simulink model "Road monito-2024r"  (R2021a)
settings: Solver=FixedStepDiscrete  StartTime=0.0  StopTime=inf  FixedStep=0.1  RelTol=1e-3
libraries: simulink x29
(part 2 of 2)

== system Road monito-2024r/rule81_2 ==
  light : Inport
  Enable : EnablePort  StatesWhenEnabling=reset
  light usage : MATLAB Function  TreatAsAtomicUnit=on
  y : Outport  OutputWhenDisabled=reset  InitialOutput=0
  wires:
  light usage/1(y) -> y/1
  light/1 -> light usage/1(light)

== system Road monito-2024r/rule81_3 ==
  Ego : Inport
  Enable : EnablePort  StatesWhenEnabling=reset
  Speedmonitor : MATLAB Function  TreatAsAtomicUnit=on
  y1 : Outport  OutputWhenDisabled=reset  InitialOutput=0
  cs : Outport  Port=2  OutputWhenDisabled=reset  InitialOutput=[0 120]
  wires:
  Speedmonitor/2(cs) -> cs/1
  Ego/1 -> Speedmonitor/1(Ego)
  Speedmonitor/1(y) -> y1/1

== system Road monito-2024r/rule81_4 ==
  Ego : Inport
  Enable : EnablePort  StatesWhenEnabling=reset
  Speedmonitor : MATLAB Function  TreatAsAtomicUnit=on
  y1 : Outport  OutputWhenDisabled=reset  InitialOutput=0
  cs : Outport  Port=2  OutputWhenDisabled=reset  InitialOutput=[0 120]
  wires:
  Speedmonitor/2(cs) -> cs/1
  Ego/1 -> Speedmonitor/1(Ego)
  Speedmonitor/1(y) -> y1/1

== system Road monito-2024r/rule81_5 ==
  Ego : Inport
  Enable : EnablePort  StatesWhenEnabling=reset
  Speedmonitor : MATLAB Function  TreatAsAtomicUnit=on
  y1 : Outport  OutputWhenDisabled=reset  InitialOutput=0
  cs : Outport  Port=2  OutputWhenDisabled=reset  InitialOutput=[0 120]
  wires:
  Speedmonitor/2(cs) -> cs/1
  Ego/1 -> Speedmonitor/1(Ego)
  Speedmonitor/1(y) -> y1/1

== system Road monito-2024r/rule81_6 ==
  Enable : EnablePort  StatesWhenEnabling=reset
  Constant : Constant  Value=100
  CD : Outport  OutputWhenDisabled=reset  InitialOutput=-1
  wires:
  Constant/1 -> CD/1

== system Road monito-2024r/rule81_7 ==
  Enable : EnablePort  StatesWhenEnabling=reset
  Constant : Constant  Value=50
  CD : Outport  OutputWhenDisabled=reset  InitialOutput=-1
  wires:
  Constant/1 -> CD/1

== system Road monito-2024r/rule82_1 ==
  Ego : Inport
  Enable : EnablePort  StatesWhenEnabling=reset
  Speedmonitor : MATLAB Function  TreatAsAtomicUnit=on
  y1 : Outport  OutputWhenDisabled=reset  InitialOutput=0
  wires:
  Ego/1 -> Speedmonitor/1(Ego)
  Speedmonitor/1(y) -> y1/1

== system Road monito-2024r/rule82_2 ==
  decision : Inport
  left1 : Inport  Port=2
  Enable : EnablePort  StatesWhenEnabling=reset
  Compare To Constant : simulink/Logic and Bit Operations/Compare To Constant  relop===  const=6  OutDataTypeStr=boolean
  Logical Operator : Logic  AllPortsSameDT=off  OutDataTypeStr=boolean
  y1 : Outport  OutputWhenDisabled=reset  InitialOutput=0
  wires:
  decision/1 -> Compare To Constant/1
  Compare To Constant/1 -> Logical Operator/1
  left1/1 -> Logical Operator/2
  Logical Operator/1 -> y1/1

== system Road monito-2024r/rule82_3 ==
  note: 待开发
  Enable : EnablePort  StatesWhenEnabling=reset
  Constant : Constant  Value=0
  y1 : Outport  OutputWhenDisabled=reset  InitialOutput=0
  wires:
  Constant/1 -> y1/1

== system Road monito-2024r/rule82_4 ==
  Ego : Inport
  Enable : EnablePort  StatesWhenEnabling=reset
  Speedmonitor : MATLAB Function  TreatAsAtomicUnit=on
  y1 : Outport  OutputWhenDisabled=reset  InitialOutput=0
  wires:
  Ego/1 -> Speedmonitor/1(Ego)
  Speedmonitor/1(y) -> y1/1

== system Road monito-2024r/rule82_5 ==
  overlap : Inport
  Enable : EnablePort  StatesWhenEnabling=reset
  Constant : Constant
  Constant1 : Constant  Value=0
  Switch : Switch  Criteria=u2 > Threshold
  y1 : Outport  OutputWhenDisabled=reset  InitialOutput=0
  wires:
  overlap/1 -> Switch/2
  Constant/1 -> Switch/1
  Constant1/1 -> Switch/3
  Switch/1 -> y1/1

== system Road monito-2024r/rule_47_2_2 ==
  T1_2_2 : Inport
  t1_2_4 : Inport  Port=2
  Ego : Inport  Port=3
  Tgtrf : Inport  Port=4
  Tgtrr : Inport  Port=5
  Enable : EnablePort  StatesWhenEnabling=reset
  Logical Operator : Logic  Operator=OR  AllPortsSameDT=off  OutDataTypeStr=boolean
  MATLAB Function : MATLAB Function  TreatAsAtomicUnit=on
  MATLAB Function1 : MATLAB Function  TreatAsAtomicUnit=on
  Out1 : Outport  OutputWhenDisabled=reset  InitialOutput=0
  wires:
  T1_2_2/1 -> MATLAB Function/1(t122)
  Ego/1 -> MATLAB Function1/2(Ego), MATLAB Function/2(Ego)
  Tgtrf/1 -> MATLAB Function/3(Tgtrf)
  t1_2_4/1 -> MATLAB Function1/1(t124)
  Tgtrr/1 -> MATLAB Function1/3(Tgtrr)
  MATLAB Function/1(y) -> Logical Operator/1
  MATLAB Function1/1(y) -> Logical Operator/2
  Logical Operator/1 -> Out1/1

== system Road monito-2024r/rule_dis ==
  Tgt_f : Inport
  Ego : Inport  Port=2
  Ego_fl : Inport  Port=3
  ycd : Inport  Port=4
  Enable : EnablePort  StatesWhenEnabling=reset
  FollowingDistance : MATLAB Function  TreatAsAtomicUnit=on
  y : Outport  OutputWhenDisabled=reset  InitialOutput=0
  wires:
  Tgt_f/1 -> FollowingDistance/2(Tgt_f)
  FollowingDistance/1(y) -> y/1
  Ego/1 -> FollowingDistance/1(Ego)
  Ego_fl/1 -> FollowingDistance/3(Ego_fl)
  ycd/1 -> FollowingDistance/4(ycd)

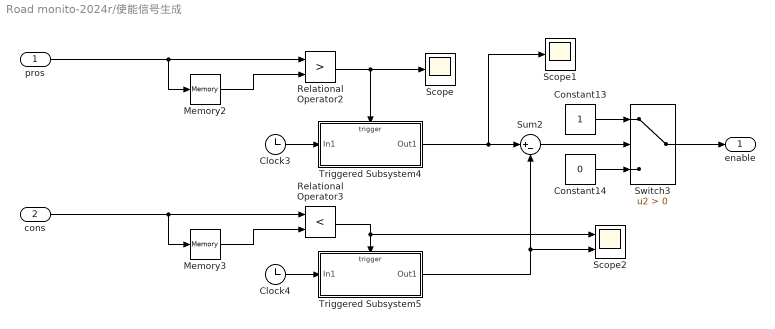
== system Road monito-2024r/使能信号生成 ==
  pros : Inport
  cons : Inport  Port=2
  Clock3 : Clock
  Clock4 : Clock
  Constant13 : Constant
  Constant14 : Constant  Value=0
  Memory2 : Memory
  Memory3 : Memory
  Relational Operator2 : RelationalOperator  Operator=>  OutDataTypeStr=boolean  RndMeth=Simplest
  Relational Operator3 : RelationalOperator  Operator=<  OutDataTypeStr=boolean  RndMeth=Simplest
  Scope : Scope
  Scope1 : Scope
  Scope2 : Scope  NumInputPorts=2
  Sum2 : Sum  Inputs=|+-
  Switch3 : Switch  Criteria=u2 > Threshold
  Triggered Subsystem4 : Subsystem  TreatAsAtomicUnit=on
  Triggered Subsystem5 : Subsystem  TreatAsAtomicUnit=on
  enable : Outport
  wires:
  Relational Operator3/1 -> Triggered Subsystem5/Trigger, Scope2/1
  Constant14/1 -> Switch3/3
  Triggered Subsystem4/1(Out1) -> Scope1/1, Sum2/1
  Sum2/1 -> Switch3/2
  pros/1 -> Memory2/1, Relational Operator2/1
  Clock4/1 -> Triggered Subsystem5/1(In1)
  Memory3/1 -> Relational Operator3/2
  Relational Operator2/1 -> Scope/1, Triggered Subsystem4/Trigger
  Memory2/1 -> Relational Operator2/2
  Clock3/1 -> Triggered Subsystem4/1(In1)
  Triggered Subsystem5/1(Out1) -> Scope2/2, Sum2/2
  Constant13/1 -> Switch3/1
  Switch3/1 -> enable/1
  cons/1 -> Memory3/1, Relational Operator3/1

== system Road monito-2024r/Enabled Subsystem/Triggered Subsystem2 ==
  In1 : Inport
  Trigger : TriggerPort  VariantControl=Variant
  Output : Outport  InitialOutput=0  VectorParamsAs1DForOutWhenUnconnected=off
  wires:
  In1/1 -> Output/1

== system Road monito-2024r/Enabled Subsystem1/Triggered Subsystem2 ==
  In1 : Inport
  Trigger : TriggerPort  VariantControl=Variant
  Output : Outport  InitialOutput=0  VectorParamsAs1DForOutWhenUnconnected=off
  wires:
  In1/1 -> Output/1

== system Road monito-2024r/Subsystem2/Enabled Subsystem1 ==
  t2_out : Inport
  roadinfo : Inport  Port=2
  Enable : EnablePort
  Selector1 : Selector  InputPortWidth=3  IndexOptions=Index vector (dialog)  Indices=[2]  OutputSizes=1
  t2 : Outport  InitialOutput=-10
  t2_laneid : Outport  Port=2  InitialOutput=0
  wires:
  t2_out/1 -> t2/1  "上一次下降沿时间"
  roadinfo/1 -> Selector1/1
  Selector1/1 -> t2_laneid/1  "上一次下降沿所在的车道"

== system Road monito-2024r/Subsystem2/Triggered Subsystem1 ==
  t1_out : Inport
  t_now : Inport  Port=2
  laneinfo : Inport  Port=3
  Trigger : TriggerPort  VariantControl=(inherit)
  t1 : Outport  InitialOutput=-20
  t3 : Outport  Port=2  InitialOutput=-10
  t1_lanid : Outport  Port=3  InitialOutput=0
  wires:
  t1_out/1 -> t1/1  "上一次上升沿时间"
  t_now/1 -> t3/1  "这一次上升沿时间"
  laneinfo/1 -> t1_lanid/1  "上一次上升沿时所在的车道"

== system Road monito-2024r/Timing module/Triggered Subsystem1 ==
  In1 : Inport
  In2 : Inport  Port=2
  Trigger : TriggerPort  TriggerType=falling  VariantControl=Variant
  Add : Sum  Inputs=-+
  Out1 : Outport  VectorParamsAs1DForOutWhenUnconnected=off
  wires:
  Add/1 -> Out1/1
  In2/1 -> Add/2
  In1/1 -> Add/1

== system Road monito-2024r/Timing module/Triggered Subsystem2 ==
  In1 : Inport
  Trigger : TriggerPort  VariantControl=Variant
  Out1 : Outport  InitialOutput=0  VectorParamsAs1DForOutWhenUnconnected=off
  wires:
  In1/1 -> Out1/1

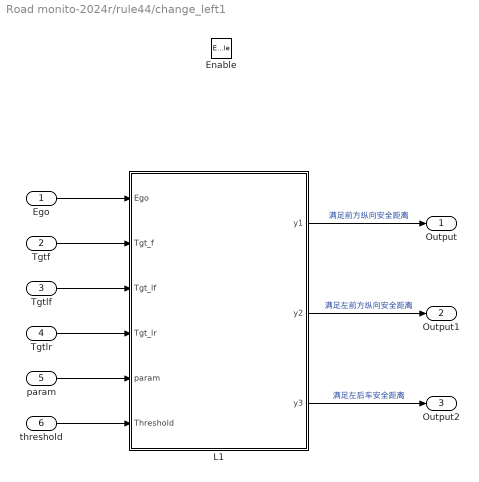
== system Road monito-2024r/rule44/change_left1 ==
  Ego : Inport
  Tgtf : Inport  Port=2
  Tgtlf : Inport  Port=3
  Tgtlr : Inport  Port=4
  param : Inport  Port=5
  threshold : Inport  Port=6
  Enable : EnablePort  StatesWhenEnabling=reset
  L1 : MATLAB Function  TreatAsAtomicUnit=on
  Output : Outport  OutputWhenDisabled=reset  InitialOutput=0
  Output1 : Outport  Port=2  OutputWhenDisabled=reset  InitialOutput=0
  Output2 : Outport  Port=3  OutputWhenDisabled=reset  InitialOutput=0
  wires:
  Ego/1 -> L1/1(Ego)
  Tgtf/1 -> L1/2(Tgt_f)
  Tgtlf/1 -> L1/3(Tgt_lf)
  Tgtlr/1 -> L1/4(Tgt_lr)
  param/1 -> L1/5(param)
  threshold/1 -> L1/6(Threshold)
  L1/1(y1) -> Output/1  "满足前方纵向安全距离"
  L1/2(y2) -> Output1/1  "满足左前方纵向安全距离"
  L1/3(y3) -> Output2/1  "满足左后车安全距离"

== system Road monito-2024r/rule44/change_left2 ==
  Ego : Inport
  Tgtf : Inport  Port=2
  Tgtr : Inport  Port=3
  param : Inport  Port=4
  threshold : Inport  Port=5
  Enable : EnablePort  StatesWhenEnabling=reset
  beforerchangelane : MATLAB Function  TreatAsAtomicUnit=on
  Output1 : Outport  OutputWhenDisabled=reset  InitialOutput=0
  Output2 : Outport  Port=2  OutputWhenDisabled=reset  InitialOutput=0
  wires:
  Ego/1 -> beforerchangelane/3(Ego)
  Tgtf/1 -> beforerchangelane/1(Tgt_f)
  Tgtr/1 -> beforerchangelane/2(Tgt_r)
  param/1 -> beforerchangelane/4(param)
  threshold/1 -> beforerchangelane/5(Threshold)
  beforerchangelane/1(y2) -> Output1/1  "满足前方纵向安全距离"
  beforerchangelane/2(y3) -> Output2/1  "满足后车安全距离"

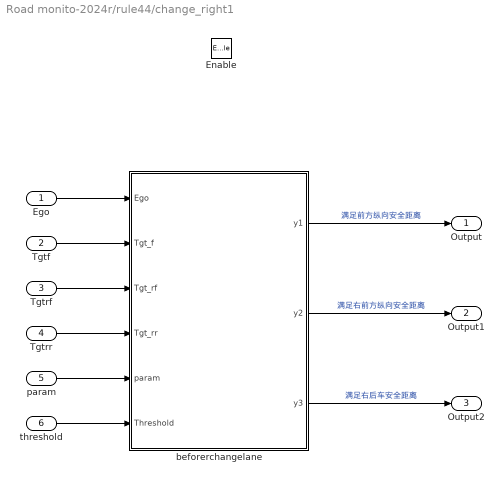
== system Road monito-2024r/rule44/change_right1 ==
  Ego : Inport
  Tgtf : Inport  Port=2
  Tgtrf : Inport  Port=3
  Tgtrr : Inport  Port=4
  param : Inport  Port=5
  threshold : Inport  Port=6
  Enable : EnablePort  StatesWhenEnabling=reset
  beforerchangelane : MATLAB Function  TreatAsAtomicUnit=on
  Output : Outport  OutputWhenDisabled=reset  InitialOutput=0
  Output1 : Outport  Port=2  OutputWhenDisabled=reset  InitialOutput=0
  Output2 : Outport  Port=3  OutputWhenDisabled=reset  InitialOutput=0
  wires:
  Ego/1 -> beforerchangelane/1(Ego)
  Tgtf/1 -> beforerchangelane/2(Tgt_f)
  Tgtrf/1 -> beforerchangelane/3(Tgt_rf)
  Tgtrr/1 -> beforerchangelane/4(Tgt_rr)
  param/1 -> beforerchangelane/5(param)
  threshold/1 -> beforerchangelane/6(Threshold)
  beforerchangelane/1(y1) -> Output/1  "满足前方纵向安全距离"
  beforerchangelane/2(y2) -> Output1/1  "满足右前方纵向安全距离"
  beforerchangelane/3(y3) -> Output2/1  "满足右后车安全距离"

== system Road monito-2024r/rule44/change_right2 ==
  Ego : Inport
  Tgtf : Inport  Port=2
  Tgtr : Inport  Port=3
  param : Inport  Port=4
  threshold : Inport  Port=5
  Enable : EnablePort  StatesWhenEnabling=reset
  beforerchangelane : MATLAB Function  TreatAsAtomicUnit=on
  Output1 : Outport  OutputWhenDisabled=reset  InitialOutput=0
  Output2 : Outport  Port=2  OutputWhenDisabled=reset  InitialOutput=0
  wires:
  Ego/1 -> beforerchangelane/3(Ego)
  Tgtf/1 -> beforerchangelane/1(Tgt_f)
  Tgtr/1 -> beforerchangelane/2(Tgt_r)
  param/1 -> beforerchangelane/4(param)
  threshold/1 -> beforerchangelane/5(Threshold)
  beforerchangelane/1(y2) -> Output1/1  "满足前方纵向安全距离"
  beforerchangelane/2(y3) -> Output2/1  "满足后车安全距离"

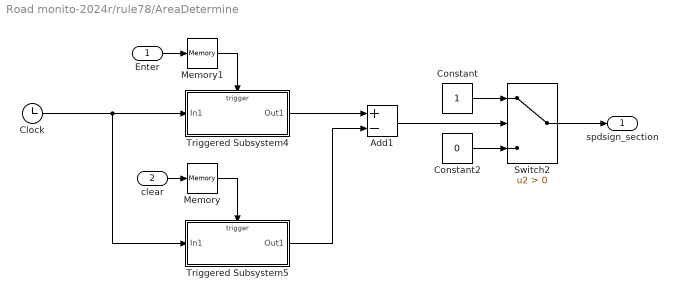
== system Road monito-2024r/rule78/AreaDetermine ==
  Enter : Inport
  clear : Inport  Port=2
  Add1 : Sum  Inputs=+-
  Clock : Clock
  Constant : Constant
  Constant2 : Constant  Value=0
  Memory : Memory
  Memory1 : Memory
  Switch2 : Switch  Criteria=u2 > Threshold
  Triggered Subsystem4 : Subsystem  TreatAsAtomicUnit=on
  Triggered Subsystem5 : Subsystem  TreatAsAtomicUnit=on
  spdsign_section : Outport
  wires:
  Triggered Subsystem4/1(Out1) -> Add1/1
  Enter/1 -> Memory1/1
  Switch2/1 -> spdsign_section/1
  clear/1 -> Memory/1
  Triggered Subsystem5/1(Out1) -> Add1/2
  Add1/1 -> Switch2/2
  Constant2/1 -> Switch2/3
  Memory/1 -> Triggered Subsystem5/Trigger
  Clock/1 -> Triggered Subsystem4/1(In1), Triggered Subsystem5/1(In1)
  Constant/1 -> Switch2/1
  Memory1/1 -> Triggered Subsystem4/Trigger

== system Road monito-2024r/使能信号生成/Triggered Subsystem4 ==
  In1 : Inport
  Trigger : TriggerPort  TriggerType=either  VariantControl=(inherit)
  Out1 : Outport
  wires:
  In1/1 -> Out1/1

== system Road monito-2024r/使能信号生成/Triggered Subsystem5 ==
  In1 : Inport
  Trigger : TriggerPort  VariantControl=(inherit)
  Out1 : Outport
  wires:
  In1/1 -> Out1/1

== system Road monito-2024r/rule78/AreaDetermine/Triggered Subsystem4 ==
  In1 : Inport
  Trigger : TriggerPort  VariantControl=(inherit)
  Out1 : Outport
  wires:
  In1/1 -> Out1/1

== system Road monito-2024r/rule78/AreaDetermine/Triggered Subsystem5 ==
  In1 : Inport
  Trigger : TriggerPort  VariantControl=(inherit)
  Out1 : Outport
  wires:
  In1/1 -> Out1/1

== matlab function Road monito-2024r/rule80/FollowingDistance ==
  data: Ego input; CD output
function CD = fcn(Ego)
%参数需求
Egovx = Ego(4);                   %自车纵向速度(m/s)

if Egovx >= 100/3.6
    CD = 100;
else
    CD = 50;
end

== matlab function Road monito-2024r/rule44/MATLAB Function ==
  data: u input; y output
function y = fcn(u)

if u == 0
    y = 0;
elseif u == 1
    y = 44.22;
elseif u == 2
    y = 44.23;
elseif u == 3
    y = 44.24;
else
    y = 0;
end

== matlab function Road monito-2024r/rule44/MATLAB Function1 ==
  data: u input; y output
function y = fcn(u)

if u == 0
    y = 0;
elseif u == 1
    y = 44.25;
elseif u == 2
    y = 44.26;
elseif u == 3
    y = 44.27;
else
    y = 0;
end

== matlab function Road monito-2024r/rule44/MATLAB Function2 ==
  data: u input; y output
function y = fcn(u)

if u == 0
    y = 0;
elseif u == 1
    y = 44.12;
elseif u == 2
    y = 44.13;
elseif u == 3
    y = 44.14;
else
    y = 0;
end

== matlab function Road monito-2024r/T_rule78 ==
  data: roadinfo input; y output
function y = fcn(roadinfo)
if roadinfo(1)==1
    y = 1;
else
    y = 0;
end

== matlab function Road monito-2024r/rule78/Speedsigncalculate ==
  data: Enter_spdlimit_section output; Ego input; speedsign input
function Enter_spdlimit_section = fcn(Ego,speedsign)
%%

%参数需求
s_speedsign = speedsign(1);         %限速标志位置(m)(感知范围内无标志则输入为2000）
Egox = Ego(1);
%高速主路限速条件判断
if s_speedsign < Egox       %限速标志检测，只用于判断是否进入限速标志管理区域
    Enter_spdlimit_section = 1;
else
    Enter_spdlimit_section = 0;
end

== matlab function Road monito-2024r/rule78/Speedmonitor ==
  data: Ego input; speedsign input; respeedsign input; spdsign_section input; y output; cs output; clear output; roadinfo input
function [y,cs,clear] = fcn(Ego,speedsign,respeedsign,spdsign_section,roadinfo)
%%

%参数需求
Ego_x = Ego(1);
Ego_vx = Ego(4);
vxmax_speedsign = speedsign(3);     %限速标志限制的速度上限(km/h)
vxmin_speedsign = speedsign(4);     %限速标志限制的速度下限(km/h)（无则输入为60）
s_releasespdsign = respeedsign(1);  %解除限速标志位置(m)(无则输入为0）
roadid = roadinfo(2);
roadnum = roadinfo(3);

%高速主路限速触发条件判断
if spdsign_section == 1       %自车处于限速标志管理路段
    if Ego_vx >= vxmin_speedsign/3.6 && Ego_vx <= vxmax_speedsign/3.6
        y = 0;
    else
        y = 1;
    end
    cs = [vxmin_speedsign vxmax_speedsign];
else                         %自车处于非限速标志管理路段
    if roadnum==2 && roadid==1
        if Ego_vx >= 100/3.6 && Ego_vx <= 120/3.6
            y = 0;
        else
            y = 1;
        end
        cs = [100 120];
    elseif roadnum>=3 && roadid==1
        if Ego_vx >= 110/3.6 && Ego_vx <= 120/3.6
            y = 0;
        else
            y = 1;
        end
        cs = [110 120];
    elseif roadnum>=3 && roadid>1 && roadid<roadnum
        if Ego_vx >= 90/3.6 && Ego_vx <= 120/3.6
            y = 0;
        else
            y = 1;
        end
        cs = [90 120];
    else
        y = 0;
        cs = [60 100];
    end
end
if s_releasespdsign < Ego_x           %解除限速标志位置，用于反馈确定自车所在区域
    clear = 1;
else
    clear = 0;
end

== matlab function Road monito-2024r/rule44/MATLAB Function3 ==
  data: u input; y output
function y = fcn(u)

if u == 0
    y = 0;
elseif u == 1
    y = 44.15;
elseif u == 2
    y = 44.16;
elseif u == 3
    y = 44.17;
else
    y = 0;
end

== matlab function Road monito-2024r/T_rule46_1 ==
  data: env input; y1 output; y2 output; y3 output
function [y1,y2,y3] = fcn(env)
if env(1)<50
    y1 = true;
    y2 = false;
    y3 = false;
elseif env(1)<100
    y1 = false;
    y2 = true;
    y3 = false;
elseif env(1)<200
    y1 = false;
    y2 = false;
    y3 = true;
else
    y1 = false;
    y2 = false;
    y3 = false;
end

== matlab function Road monito-2024r/rule46_1/Speedmonitor ==
  data: Ego input; y output; cs output
function [y,cs] = fcn(Ego)
%%

%参数需求
Ego_vx = Ego(4);


if Ego_vx <= 30/3.6
    y = 0;
else
    y = 1;
end
cs = [0 30];

== matlab function Road monito-2024r/T_rule46_2 ==
  data: env input; y output
function y = fcn(env)
if env(2)==1
    y = 1;
else
    y = 0;
end

== matlab function Road monito-2024r/rule46_2/Speedmonitor ==
  data: Ego input; y output; cs output
function [y,cs] = fcn(Ego)
%%

%参数需求
Ego_vx = Ego(4);


if Ego_vx <= 30/3.6
    y = 0;
else
    y = 1;
end
cs = [0 30];

== matlab function Road monito-2024r/rule44/change_right1/beforerchangelane ==
  data: Ego input; Tgt_f input; Tgt_rf input; Tgt_rr input; y1 output; y2 output; y3 output; param input; Threshold input
function [y1,y2,y3] = fcn(Ego,Tgt_f,Tgt_rf,Tgt_rr,param,Threshold)
%%

%参数需求

Tgtx_rr = Tgt_rr(1);             
Tgty_rr = Tgt_rr(2);              
Tgtvx_rr = Tgt_rr(3);
Tgtl_rr = Tgt_rr(5);
Egox = Ego(1);
Egovx = Ego(4);
Egol = param(1);
Ego_fl = param(3);
Tgtx_f = Tgt_f(1);              
Tgty_f = Tgt_f(2);
Tgtvx_f = Tgt_f(3);
Tgtl_f = Tgt_f(5);
Tgtx_rf = Tgt_rf(1);              
Tgty_rf = Tgt_rf(2);
Tgtvx_rf = Tgt_rf(3); 
Tgtl_rf = Tgt_rf(5);
dclmin = Threshold(9) * (Egovx - Tgtvx_rr) + Threshold(10);         %最小换道距离
if dclmin > 50
    dclmin = 50;
elseif dclmin < 0
    dclmin = 0;
else
    dclmin = dclmin;
end
TTCx = Threshold(3);           %安全碰撞时间

%与前车的安全距离判断
if Tgtx_f == 2000 && Tgty_f == 2000       %坐标为2000视为不存在前车
    y1 = 0;   
else
    if Tgtx_f-Egox-0.5*Tgtl_f-Ego_fl < (Egovx - Tgtvx_f) * TTCx 
        y1 = 1;
%     elseif Tgtx_f-Egox-0.5*Tgtl_f-Ego_fl < dclmin %前车暂不考虑车距
%         y1 = 2;
    else
        y1 = 0;
    end
end
%与右前车的安全距离判断
if Tgtx_rf == 2000 && Tgty_rf == 2000     %坐标为2000视为不存在右前车
    y2 = 0;
else
    if Tgtx_rf-Egox-0.5*Tgtl_rf-Ego_fl < (Egovx - Tgtvx_rf) * TTCx 
        y2 = 1;
    else
        y2 = 0;
    end
end
%与右后车的安全距离判断
if Tgtx_rr == 2000 && Tgty_rr == 2000   %坐标为2000视为不存在右后车
    y3 = 0;
else
    if Egox-Tgtx_rr-0.5*Tgtl_rr-(Egol-Ego_fl) < dclmin
        y3 = 3;
    else
        y3 = 0;
    end
end

== matlab function Road monito-2024r/rule47_1_l/Speedmonitor ==
  data: threshold input; light input; y output
function y = fcn(threshold,light)
%%
t_cl = threshold(4);

if light >= t_cl
    y = 0;
else
    y = 1;
end

== matlab function Road monito-2024r/rule47_1_r/Speedmonitor ==
  data: threshold input; light input; y output
function y = fcn(threshold,light)
%%
t_cl = threshold(4);

if light >= t_cl
    y = 0;
else
    y = 1;
end

== matlab function Road monito-2024r/rule1_43/MATLAB Function ==
  data: Tgtf input; y output; left input
function y = fcn(Tgtf,left)

Tgtfx = Tgtf(1);
Tgtfy = Tgtf(2);
Tgtfvy = Tgtf(4);
Tgtfw = Tgtf(6);

yTgt_l = Tgtfy + 0.5 * Tgtfw;
yTgt_r = Tgtfy - 0.5 * Tgtfw;

Y_leftline_Ego = polyval(left(2:end-1),Tgtfx);

if Y_leftline_Ego<yTgt_l && Y_leftline_Ego>yTgt_r
    y1 = 1;
else
    y1 = 0;
end

if Tgtfvy > 0.2
    y2 = 1;
else
    y2 = 0;
end

if y1==1 && y2 ==1
    y = 1;
else
    y = 0;
end

== matlab function Road monito-2024r/T_overlapline ==
  data: param input; left input; right input; y output
function y = fcn(param,left,right)

Ego_l = param(1);
Ego_w = param(2);
Ego_fl = param(3);

yEgo_lf = 0.5 * Ego_w;
yEgo_rf = -0.5 * Ego_w;
yEgo_lr = 0.5 * Ego_w;
yEgo_rr = -0.5 * Ego_w;

Y_leftline_Egof = polyval(left(2:end-1),Ego_fl);
Y_leftline_Egor = polyval(left(2:end-1),Ego_fl - Ego_l);
Y_rightline_Egof = polyval(right(2:end-1),Ego_fl);
Y_rightline_Egor = polyval(right(2:end-1),Ego_fl - Ego_l);

if Y_leftline_Egof<yEgo_lf && Y_leftline_Egof>yEgo_rf
    y = 1;
elseif Y_rightline_Egof<yEgo_lf && Y_rightline_Egof>yEgo_rf
    y = 2;
elseif Y_leftline_Egor<yEgo_lr && Y_leftline_Egor>yEgo_rr
    y = 1;
elseif Y_rightline_Egor<yEgo_lr && Y_rightline_Egor>yEgo_rr
    y = 2;
else
    y = 0;
end

== matlab function Road monito-2024r/rule1_43/MATLAB Function1 ==
  data: Tgtlf input; y output; left input
function y = fcn(Tgtlf,left)

Tgtlfx = Tgtlf(1);
Tgtlfy = Tgtlf(2);
Tgtlfvy = Tgtlf(4);
Tgtlfw = Tgtlf(6);

yTgt_l = Tgtlfy + 0.5 * Tgtlfw;
yTgt_r = Tgtlfy - 0.5 * Tgtlfw;

Y_leftline_Ego = polyval(left(2:end-1),Tgtlfx);

if Y_leftline_Ego<yTgt_l && Y_leftline_Ego>yTgt_r
    y1 = 1;
else
    y1 = 0;
end

if Tgtlfvy > 0.2
    y2 = 1;
else
    y2 = 0;
end

if y1==1 && y2 ==1
    y = 1;
else
    y = 0;
end

== matlab function Road monito-2024r/rule_47_2_2/MATLAB Function ==
  data: t122 input; y output; Ego input; Tgtrf input
function y = fcn(t122,Ego,Tgtrf)

if t122 == 0
    y = 0;
else
    if Ego(4) - Tgtrf(3) > 15/3.6
        y = 0;
    else
        y = 1;
    end
end

== matlab function Road monito-2024r/rule_47_2_2/MATLAB Function1 ==
  data: t124 input; y output; Ego input; Tgtrr input
function y = fcn(t124,Ego,Tgtrr)

if t124 == 0
    y = 0;
else
    if Ego(4) - Tgtrr(3) > 15/3.6
        y = 0;
    else
        y = 1;
    end
end

== matlab function Road monito-2024r/rule1_43/MATLAB Function2 ==
  data: specsec input; y output
function y = fcn(specsec)

if specsec(1)==1 || specsec(2)==1
    y = 1;
else
    y = 0;
end

== matlab function Road monito-2024r/rule79_3/light usage ==
  data: light input; y output
function y = fcn(light)


if light(2)==1
    y = 0;
else
    y = 1;
end

== matlab function Road monito-2024r/MATLAB Function6 ==
  data: cs1 input; ycs output; cs2 input; cs3 input; cs4 input; cs5 input; cs6 input
function ycs = fcn(cs1,cs2,cs3,cs4,cs5,cs6)

cs_1 = [cs1(1),cs2(1),cs3(1),cs4(1),cs5(1),cs6(1)];
cs_2 = [cs1(2),cs2(2),cs3(2),cs4(2),cs5(2),cs6(2)];
csup = min(cs_2);

flag = cs_1 < csup;
cslow = max(cs_1(flag));

ycs = [cslow csup];

== matlab function Road monito-2024r/rule80/FollowingDistance1 ==
  data: y output; Ego input; Tgt_f input; Dis output; Ego_fl input; CD output
function [y,Dis,CD] = fcn(Ego,Tgt_f, Ego_fl)
%参数需求
Tgtx_f = Tgt_f(1);              %超车目标纵坐标(m)
Tgtl_f = Tgt_f(5);
Egox = Ego(1);                    %自车纵坐标（）
Egovx = Ego(4);                   %自车纵向速度(m/s)

if Egovx >= 100/3.6
    if Tgtx_f-Egox-Ego_fl-0.5*Tgtl_f >100
        y = 0;
    else
        y = 1;
    end
    CD = 100;
else
    if Tgtx_f-Egox-Ego_fl-0.5*Tgtl_f >50
        y = 0;
    else
        y = 1;
    end
    CD = 50;
end
Dis = Tgtx_f-Egox-Ego_fl-0.5*Tgtl_f;

== matlab function Road monito-2024r/zoning ==
  data: Ego input; Tgt_f output; Tgt_x input; Tgt_y input; Tgt_vx input; Tgt_vy input; Tgt_l input; Tgt_w input; Tgt_r output; Tgt_lf output; Tgt_lr output; Tgt_rf output; Tgt_rr output; nextleft input; left input; right input; nextright input
function [Tgt_f,Tgt_r,Tgt_lf,Tgt_lr,Tgt_rf,Tgt_rr] = fcn(Ego,Tgt_x,Tgt_y,Tgt_vx,Tgt_vy,Tgt_l,Tgt_w,nextleft,left,right,nextright)

Ego_x = Ego(1);
%若他车不存在，则输入全为0

%车道线宽度
w_lane = polyval(left(2:end-1),0) - polyval(right(2:end-1),0);

%方位分割
Flag = abs(Tgt_x) > 0.1 | abs(Tgt_y) > 0.1;  %剔除不存在车辆
Flag1 = Tgt_x > Ego_x;      %他车位于自车之前
Flag2 = Tgt_x <= Ego_x;     %他车位于自车之后

if nextleft(1) == -1        %自车位于最左侧车道
    Flag3 = (Tgt_y>=polyval(right(2:end-1),Tgt_x) & Tgt_y<polyval(left(2:end-1),Tgt_x));      %同车道他车
    Flag5 = false(1,20);    %左侧车道他车
    if nextright(1) == 0	%右侧车道他车
        Flag4 = (Tgt_y>=polyval(right(2:end-1),Tgt_x)-w_lane & Tgt_y<polyval(right(2:end-1),Tgt_x));
    elseif nextright(1) == -1
        Flag4 = false(1,20);
    else
        Flag4 = (Tgt_y>=polyval(nextright(2:end-1),Tgt_x) & Tgt_y<polyval(right(2:end-1),Tgt_x));
    end
elseif nextright(1) == -1  %自车位于最右侧车道
    Flag3 = (Tgt_y>=polyval(right(2:end-1),Tgt_x) & Tgt_y<polyval(left(2:end-1),Tgt_x));      %同车道他车
    Flag4 = false(1,20);  %右侧车道他车
    if nextleft(1) == 0   %左侧车道他车
        Flag5 = (Tgt_y>=polyval(left(2:end-1),Tgt_x) & Tgt_y<polyval(left(2:end-1),Tgt_x)+w_lane); 
    elseif nextleft(1) == -1
        Flag5 = false(1,20);
    else
        Flag5 = (Tgt_y>=polyval(left(2:end-1),Tgt_x) & Tgt_y<polyval(nextleft(2:end-1),Tgt_x));
    end
else
    Flag3 = (Tgt_y>=polyval(right(2:end-1),Tgt_x) & Tgt_y<polyval(left(2:end-1),Tgt_x));      %同车道他车
    if nextleft(1) == 0   %左侧车道他车
        Flag5 = (Tgt_y>=polyval(left(2:end-1),Tgt_x) & Tgt_y<polyval(left(2:end-1),Tgt_x)+w_lane); 
    else
        Flag5 = (Tgt_y>=polyval(left(2:end-1),Tgt_x) & Tgt_y<polyval(nextleft(2:end-1),Tgt_x));
    end
    if nextright(1) == 0  %右侧车道他车
        Flag4 = (Tgt_y>=polyval(right(2:end-1),Tgt_x)-w_lane & Tgt_y<polyval(right(2:end-1),Tgt_x));
    else
        Flag4 = (Tgt_y>=polyval(nextright(2:end-1),Tgt_x) & Tgt_y<polyval(right(2:end-1),Tgt_x));
    end
end
%筛选六个方位中离自车最近的车，即每个方位区域只保留一辆车
Flag_f = Flag & Flag1 & Flag3;      %同车道前车
if any(Flag_f)
    f_min = min(abs(Tgt_x(Flag_f) - Ego_x));
    Tgt_x_f = (sign(min(Tgt_x(Flag_f) - Ego_x)) * f_min) + Ego_x;
    col_f = find(abs(Tgt_x-Tgt_x_f)<=0.0001 & Flag_f == true);
    if ~isempty(col_f)
        Tgt_y_f = Tgt_y(col_f(1));
        Tgt_vx_f = Tgt_vx(col_f(1));
        Tgt_vy_f = Tgt_vy(col_f(1));
        Tgt_l_f = Tgt_l(col_f(1));
        Tgt_w_f = Tgt_w(col_f(1));
    else
        Tgt_y_f = 2000;
        Tgt_vx_f = 2000;
        Tgt_vy_f = 2000;
        Tgt_l_f = 2000;
        Tgt_w_f = 2000;
    end
else
    f_min = 0;
    Tgt_x_f = 2000;
    Tgt_y_f = 2000;
    Tgt_vx_f = 2000;
    Tgt_vy_f = 2000;
    Tgt_l_f = 2000;
    Tgt_w_f = 2000;
end
Tgt_f = [Tgt_x_f, Tgt_y_f, Tgt_vx_f, Tgt_vy_f, Tgt_l_f, Tgt_w_f];

Flag_b = Flag & Flag2 & Flag3;      %同车道后车
if any(Flag_b)
    b_min = min(abs(Tgt_x(Flag_b) - Ego_x));
    Tgt_x_b = (sign(min(Tgt_x(Flag_b) - Ego_x)) * b_min) + Ego_x;
    col_b = find(abs(Tgt_x-Tgt_x_b)<=0.0001 & Flag_b == true);
    if ~isempty(col_b)
        Tgt_y_b = Tgt_y(col_b(1));
        Tgt_vx_b = Tgt_vx(col_b(1));
        Tgt_vy_b = Tgt_vy(col_b(1));
        Tgt_l_b = Tgt_l(col_b(1));
        Tgt_w_b = Tgt_w(col_b(1));
    else
        Tgt_y_b = 2000;
        Tgt_vx_b = 2000;
        Tgt_vy_b = 2000;
        Tgt_l_b = 2000;
        Tgt_w_b = 2000;
    end
else
    b_min = 0;
    Tgt_x_b = 2000;
    Tgt_y_b = 2000;
    Tgt_vx_b = 2000;
    Tgt_vy_b = 2000;
    Tgt_l_b = 2000;
    Tgt_w_b = 2000;
end
Tgt_r = [Tgt_x_b, Tgt_y_b, Tgt_vx_b, Tgt_vy_b, Tgt_l_b, Tgt_w_b];

Flag_lf = (Flag & Flag1 & Flag5);     %左侧车道前车
if any(Flag_lf)
    lf_min = min(abs(Tgt_x(Flag_lf) - Ego_x));
    Tgt_x_lf = (sign(min(Tgt_x(Flag_lf) - Ego_x)) * lf_min) + Ego_x;
    col_lf = find(abs(Tgt_x-Tgt_x_lf)<=0.0001 & Flag_lf == true);
    if ~isempty(col_lf)
        Tgt_y_lf = Tgt_y(col_lf(1));
        Tgt_vx_lf = Tgt_vx(col_lf(1));
        Tgt_vy_lf = Tgt_vy(col_lf(1));
        Tgt_l_lf = Tgt_l(col_lf(1));
        Tgt_w_lf = Tgt_w(col_lf(1));
    else
        Tgt_y_lf = 2000;
        Tgt_vx_lf = 2000;
        Tgt_vy_lf = 2000;
        Tgt_l_lf = 2000;
        Tgt_w_lf = 2000;
    end
else
    lf_min = 0;
    Tgt_x_lf = 2000;
    Tgt_y_lf = 2000;
    Tgt_vx_lf = 2000;
    Tgt_vy_lf = 2000;
    Tgt_l_lf = 2000;
    Tgt_w_lf = 2000;
end
Tgt_lf = [Tgt_x_lf, Tgt_y_lf, Tgt_vx_lf, Tgt_vy_lf, Tgt_l_lf, Tgt_w_lf];

Flag_lr = Flag & Flag2 & Flag5;     %左侧车道后车
if any(Flag_lr)
    lr_min = min(abs(Tgt_x(Flag_lr) - Ego_x));
    Tgt_x_lr = (sign(min(Tgt_x(Flag_lr) - Ego_x)) * lr_min) + Ego_x;
    col_lr = find(abs(Tgt_x-Tgt_x_lr)<=0.0001 & Flag_lr == true);
    if ~isempty(col_lr)
        Tgt_y_lr = Tgt_y(col_lr(1));
        Tgt_vx_lr = Tgt_vx(col_lr(1));
        Tgt_vy_lr = Tgt_vy(col_lr(1));
        Tgt_l_lr = Tgt_l(col_lr(1));
        Tgt_w_lr = Tgt_w(col_lr(1));
    else
        Tgt_y_lr = 2000;
        Tgt_vx_lr = 2000;
        Tgt_vy_lr = 2000;
        Tgt_l_lr = 2000;
        Tgt_w_lr = 2000;
    end
else
    lr_min = 0;
    Tgt_x_lr= 2000;
    Tgt_y_lr = 2000;
    Tgt_vx_lr = 2000;
    Tgt_vy_lr = 2000;
    Tgt_l_lr = 2000;
    Tgt_w_lr = 2000;
end
Tgt_lr = [Tgt_x_lr, Tgt_y_lr, Tgt_vx_lr, Tgt_vy_lr, Tgt_l_lr, Tgt_w_lr];

Flag_rf = Flag & Flag1 & Flag4;     %右侧车道前车
if any(Flag_rf)
    rf_min = min(abs(Tgt_x(Flag_rf) - Ego_x));
    Tgt_x_rf = (sign(min(Tgt_x(Flag_rf) - Ego_x)) * rf_min) + Ego_x;
    col_rf = find(abs(Tgt_x-Tgt_x_rf)<=0.0001 & Flag_rf == true);
    if ~isempty(col_rf)
        Tgt_y_rf = Tgt_y(col_rf(1));
        Tgt_vx_rf = Tgt_vx(col_rf(1));
        Tgt_vy_rf = Tgt_vy(col_rf(1));
        Tgt_l_rf = Tgt_l(col_rf(1));
        Tgt_w_rf = Tgt_w(col_rf(1));
    else
        Tgt_y_rf = 2000;
        Tgt_vx_rf = 2000;
        Tgt_vy_rf = 2000;
        Tgt_l_rf = 2000;
        Tgt_w_rf = 2000;
    end
else
    rf_min = 0;
    Tgt_x_rf = 2000;
    Tgt_y_rf = 2000;
    Tgt_vx_rf = 2000;
    Tgt_vy_rf = 2000;
    Tgt_l_rf = 2000;
    Tgt_w_rf = 2000;
end
Tgt_rf = [Tgt_x_rf, Tgt_y_rf, Tgt_vx_rf, Tgt_vy_rf, Tgt_l_rf, Tgt_w_rf];

Flag_rr = Flag & Flag2 & Flag4;     %同车道后车
if any(Flag_rr)
    rr_min = min(abs(Tgt_x(Flag_rr) - Ego_x));
    Tgt_x_rr = (sign(min(Tgt_x(Flag_rr) - Ego_x)) * rr_min) + Ego_x;
    col_rr = find(abs(Tgt_x-Tgt_x_rr)<=0.0001 & Flag_rr == true);
    if ~isempty(col_rr)
        Tgt_y_rr = Tgt_y(col_rr(1));
        Tgt_vx_rr = Tgt_vx(col_rr(1));
        Tgt_vy_rr = Tgt_vy(col_rr(1));
        Tgt_l_rr = Tgt_l(col_rr(1));
        Tgt_w_rr = Tgt_w(col_rr(1));
    else
        Tgt_y_rr = 2000;
        Tgt_vx_rr = 2000;
        Tgt_vy_rr = 2000;
        Tgt_l_rr = 2000;
        Tgt_w_rr = 2000;
    end
else
    rr_min = 0;
    Tgt_x_rr = 2000;
    Tgt_y_rr = 2000;
    Tgt_vx_rr = 2000;
    Tgt_vy_rr = 2000;
    Tgt_l_rr = 2000;
    Tgt_w_rr = 2000;
end
Tgt_rr = [Tgt_x_rr, Tgt_y_rr, Tgt_vx_rr, Tgt_vy_rr, Tgt_l_rr, Tgt_w_rr];

== matlab function Road monito-2024r/rule_dis/FollowingDistance ==
  data: y output; Ego input; Tgt_f input; Ego_fl input; ycd input
function y = fcn(Ego,Tgt_f, Ego_fl, ycd)
%参数需求
Tgtx_f = Tgt_f(1);              
Tgtl_f = Tgt_f(5);
Egox = Ego(1);                    

if Tgtx_f-Egox-Ego_fl-0.5*Tgtl_f > ycd
    y = 0;
else
    y = 1;
end

== matlab function Road monito-2024r/MATLAB Function7 ==
  data: Ego input; y output; ycs input
function y = fcn(Ego, ycs)

Egovx = Ego(4);

if Egovx >= ycs(1)/3.6 && Egovx <= ycs(2)/3.6
    y = 0;
else
    y = 1;
end

== matlab function Road monito-2024r/Subsystem2/MATLAB Function3 ==
  data: roadinfo input; t input; u input; y output; throshold input
function y   = get_time(roadinfo, t, u, throshold)

laneid = roadinfo(2);
cl_gap = throshold(6);
persistent last_start_time last_start_id last_end_time last_end_id start_time start_id end_time end_id;

if isempty(last_start_time) || isempty(last_start_id) || isempty(last_end_time) || isempty(last_end_id) ...
    || isempty(start_time) || isempty(start_id) || isempty(end_time) || isempty(end_id)
    last_start_time = -20;
    last_start_id = 0;
    last_end_time = -10;
    last_end_id = 0;
    start_time = 0;
    start_id = 0;
    end_time = 0;
    end_id = 0;
end

if u > 0  % 上升沿，计算本次上升沿时间与上次成功换道下降沿的时间差
    start_time = t;
    start_id = laneid;
    if start_time - last_end_time >= cl_gap
        y = 0;
    else
        y = 1;
    end
elseif u < 0  % 下降沿，根据本次换道起始id与结束id判断是否成功换道，更新数据
    y = 0;
    end_time = t;
    end_id = laneid;
    if start_id ~= end_id % 属于成功换道，更新last数据
        last_start_time = start_time;
        last_end_time = end_time;
    end
else
    y = 0;
end

end

== matlab function Road monito-2024r/Subsystem2/MATLAB Function4 ==
  data: roadinfo input; t input; u input; t1_out output; l1_out output
function [t1_out,l1_out]  = get_time(roadinfo,t, u)

laneid = roadinfo(2);
persistent t1 l1;

if isempty(t1) || isempty(l1)
    t1 = -20;
    l1 = 0;
end

if u > 0  % 上升沿
    t1_out = t1;
    l1_out = l1;
    t1 = t;
    l1 = laneid;
else
    t1_out = 0;
    l1_out = 0;
end

end

== matlab function Road monito-2024r/Subsystem2/MATLAB Function5 ==
  data: u1 input; y output; u1delay input
function y = fcn(u1,u1delay)

if u1 > u1delay % 上升沿，开始换道
    y = 1;
elseif u1 < u1delay % 下降沿，结束换道
    y = -1;
else
    y = 0;
end

== matlab function Road monito-2024r/T_rule53_1 ==
  data: Ego input; Tgt_f input; y output; Tgtx input; Tgtvx input
function y = fcn(Ego,Tgt_f,Tgtx,Tgtvx)

%参数需求
Egovx = Ego(4);
Tgtx_f = Tgt_f(1);              

flag = Tgtx~=0;
averagevx = (sum(Tgtvx(flag))+Egovx)/(length(Tgtvx(flag))+1);

%与前车的安全距离判断
if Tgtx_f ~= 2000 && averagevx < 50/3.6
    y = 1;   
else
    y = 0;
end

== matlab function Road monito-2024r/T_rule58_1 ==
  data: env input; y output
function y = fcn(env)
if env(3)==1 || env(1)<200
    y = 1;
else
    y = 0;
end

== matlab function Road monito-2024r/rule58_1/light usage ==
  data: light input; y output
function y = fcn(light)


if any(~light(6:8))
    y = 1;
else
    y = 0;
end

== matlab function Road monito-2024r/T_rule79_3 ==
  data: roadinfo input; y output; dec input
function y = fcn(roadinfo,dec)
if roadinfo(1)==1 && roadinfo(2)==roadinfo(3) && dec==2
    y = 1;
else
    y = 0;
end

== matlab function Road monito-2024r/rule58_2/light usage ==
  data: light input; y output
function y = fcn(light)


if light(4)==1
    y = 1;
else
    y = 0;
end

== matlab function Road monito-2024r/T_rule58_2 ==
  data: Ego input; Tgt_f input; y output; param input
function y = fcn(Ego,Tgt_f,param)
%%

%参数需求

Egox = Ego(1);
Ego_fl = param(3);
Tgtx_f = Tgt_f(1);              
Tgtl_f = Tgt_f(5);

%与前车的安全距离判断
if Tgtx_f ~= 2000 && Tgtx_f-Egox-0.5*Tgtl_f-Ego_fl < 50
    y = 1;   
else
    y = 0;
end

== matlab function Road monito-2024r/T_rule79_4 ==
  data: roadinfo input; y output
function y = fcn(roadinfo)
if roadinfo(1)==4
    y = 1;
else
    y = 0;
end

== matlab function Road monito-2024r/T_rule79_1 ==
  data: roadinfo input; y output; dec input
function y = fcn(roadinfo,dec)
if roadinfo(1)==3 && dec==1
    y = 1;
else
    y = 0;
end

== matlab function Road monito-2024r/rule79_1/light usage ==
  data: light input; y output
function y = fcn(light)


if light(1)==1
    y = 0;
else
    y = 1;
end

== matlab function Road monito-2024r/T_rule79_2 ==
  data: roadinfo input; y output; dec input
function y = fcn(roadinfo,dec)
if roadinfo(1)==3 && dec==1
    y = 1;
else
    y = 0;
end

== matlab function Road monito-2024r/rule79_4/MATLAB Function ==
  data: Ego input; y output; threshold input
function y = fcn(Ego,threshold)

Egovx = Ego(4);
Egoax = Ego(6);
ramp_tgtvx = threshold(5);

if Egovx < ramp_tgtvx/3.6 || Egoax < (ramp_tgtvx/3.6-Egovx)/5
    y = 0;
else
    y = 1;
end

== matlab function Road monito-2024r/rule81_3/Speedmonitor ==
  data: Ego input; y output; cs output
function [y,cs] = fcn(Ego)
%%

%参数需求
Ego_vx = Ego(4);


if Ego_vx <= 60/3.6
    y = 0;
else
    y = 1;
end
cs = [0 60];

== matlab function Road monito-2024r/rule81_1/light usage ==
  data: light input; y output
function y = fcn(light)

if any(~light([3,5:8]))
    y = 1;
else
    y = 0;
end

== matlab function Road monito-2024r/rule81_2/light usage ==
  data: light input; y output
function y = fcn(light)

if any(~light([3,5:9]))
    y = 1;
else
    y = 0;
end

== matlab function Road monito-2024r/rule81_4/Speedmonitor ==
  data: Ego input; y output; cs output
function [y,cs] = fcn(Ego)
%%

%参数需求
Ego_vx = Ego(4);


if Ego_vx <= 40/3.6
    y = 0;
else
    y = 1;
end
cs = [0 40];

== matlab function Road monito-2024r/rule81_5/Speedmonitor ==
  data: Ego input; y output; cs output
function [y,cs] = fcn(Ego)
%%

%参数需求
Ego_vx = Ego(4);


if Ego_vx <= 20/3.6
    y = 0;
else
    y = 1;
end
cs = [0 20];

== matlab function Road monito-2024r/Subsystem2/MATLAB Function6 ==
  data: throshold input; t_gap input; y output
function y = fcn(throshold,t_gap)

cl_gap = throshold(6);

if t_gap > cl_gap || t_gap < 0
    y = 0;
else
    y = 1;
end

== matlab function Road monito-2024r/rule82_1/Speedmonitor ==
  data: Ego input; y output
function y = fcn(Ego)
%%

%参数需求
Ego_vx = Ego(4);


if Ego_vx < 0
    y = 1;
else
    y = 0;
end

== matlab function Road monito-2024r/T_rule79_5 ==
  data: roadinfo input; y output
function y = fcn(roadinfo)
if roadinfo(1)==2 || roadinfo(1)==3 || roadinfo(1)==4
    y = 1;
else
    y = 0;
end

== matlab function Road monito-2024r/MATLAB Function ==
  data: roadinfo input; y output
function y = fcn(roadinfo)

if roadinfo(2)==1
    y = 1;
else
    y = 0;
end

== matlab function Road monito-2024r/rule82_4/Speedmonitor ==
  data: Ego input; y output
function y = fcn(Ego)
%%

%参数需求
Ego_vx = Ego(4);


if Ego_vx == 0
    y = 1;
else
    y = 0;
end

== matlab function Road monito-2024r/MATLAB Function1 ==
  data: Tgtlf input; y output; param input; Ego input
function y = fcn(Tgtlf,param,Ego)

tgtx = Tgtlf(1);
tgtl = Tgtlf(5);
Egox = Ego(1);
Egofl = param(3);

if tgtx-0.5*tgtl < Egox+Egofl
    y = 1;
else
    y = 0;
end

== matlab function Road monito-2024r/isexistTgt_f ==
  data: Tgt_f input; y output
function y = fcn(Tgt_f)
Tgtx_f = Tgt_f(1);              %前车纵坐标(m)
Tgty_f = Tgt_f(2);              %前车横坐标(m)

if Tgtx_f ~=2000 && Tgty_f ~=2000     %坐标不为0视为存在前车
    y = 1;
else
    y = 0;
end

== matlab function Road monito-2024r/rule1_2_1/LatDis ==
  data: Tgtlf input; y output; param input; Ego input
function y = fcn(Tgtlf,param,Ego)

tgty = Tgtlf(2);
tgtw = Tgtlf(6);
Egoy = Ego(2);
Egow = param(2);

if tgty-0.5*tgtw-Egoy-0.5*Egow > 1.5
    y = 0;
else
    y = 1;
end

== matlab function Road monito-2024r/MATLAB Function2 ==
  data: Tgtrf input; y output; param input; Ego input
function y = fcn(Tgtrf,param,Ego)

tgtx = Tgtrf(1);
tgtl = Tgtrf(5);
Egox = Ego(1);
Egofl = param(3);

if tgtx-0.5*tgtl < Egox+Egofl
    y = 1;
else
    y = 0;
end

== matlab function Road monito-2024r/rule1_2_2/LatDis ==
  data: Tgtrf input; y output; param input; Ego input
function y = fcn(Tgtrf,param,Ego)

tgty = Tgtrf(2);
tgtw = Tgtrf(6);
Egoy = Ego(2);
Egow = param(2);

if -tgty-0.5*tgtw-Egoy-0.5*Egow > 1.5
    y = 0;
else
    y = 1;
end

== matlab function Road monito-2024r/MATLAB Function3 ==
  data: Tgtlr input; y output; param input; Ego input
function y = fcn(Tgtlr,param,Ego)

tgtx = Tgtlr(1);
tgtl = Tgtlr(5);
Egox = Ego(1);
Egofl = param(3);
Egol = param(1);

if tgtx == 2000 && tgtl == 2000
    y = 0;
elseif tgtx+0.5*tgtl > Egox+Egofl-Egol
    y = 1;
else
    y = 0;
end

== matlab function Road monito-2024r/MATLAB Function4 ==
  data: Tgtrr input; y output; param input; Ego input
function y = fcn(Tgtrr,param,Ego)

tgtx = Tgtrr(1);
tgtl = Tgtrr(5);
Egox = Ego(1);
Egofl = param(3);
Egol = param(1);
if tgtx == 2000 && tgtl == 2000
    y = 0;
elseif tgtx+0.5*tgtl > Egox+Egofl-Egol
    y = 1;
else
    y = 0;
end

== matlab function Road monito-2024r/rule1_2_3/LatDis ==
  data: Tgtlr input; y output; param input; Ego input
function y = fcn(Tgtlr,param,Ego)

tgty = Tgtlr(2);
tgtw = Tgtlr(6);
Egoy = Ego(2);
Egow = param(2);

if tgty-0.5*tgtw-Egoy-0.5*Egow > 1.5
    y = 0;
else
    y = 1;
end

== matlab function Road monito-2024r/rule1_2_4/LatDis ==
  data: Tgtrr input; y output; param input; Ego input
function y = fcn(Tgtrr,param,Ego)

tgty = Tgtrr(2);
tgtw = Tgtrr(6);
Egoy = Ego(2);
Egow = param(2);

if -tgty-0.5*tgtw-Egoy-0.5*Egow > 1.5
    y = 0;
else
    y = 1;
end

== matlab function Road monito-2024r/rule79_5/MATLAB Function ==
  data: Ego input; y output; threshold input
function y = fcn(Ego,threshold)

Egovx = Ego(4);
Egoax = Ego(6);
construction_tgtvx = threshold(8);

if Egovx < construction_tgtvx/3.6 || Egoax < (construction_tgtvx/3.6-Egovx)/5
    y = 0;
else
    y = 1;
end

== matlab function Road monito-2024r/MATLAB Function5 ==
  data: initiallane input; laneid input; y output
function y = fcn(initiallane,laneid)

if laneid == initiallane
    y = 0;
elseif laneid < initiallane
    y = -1;
else
    y = 1;
end

== matlab function Road monito-2024r/T_rule1_1 ==
  data: Ego input; Tgt_f input; y output; param input; cs input
function y = fcn(Ego,Tgt_f,param,cs)

%参数需求
Egox = Ego(1);
Ego_fl = param(3);
Tgtx_f = Tgt_f(1); 
Tgtvx_f = Tgt_f(3);
Tgtl_f = Tgt_f(5);

%与前车的安全距离判断
if Tgtx_f ~= 2000 && Tgtvx_f>cs(1)/3.6 && Tgtvx_f<cs(2)/3.6
    y = 1;   
else
    y = 0;
end

== matlab function Road monito-2024r/rule1_1/speed consistent ==
  data: Ego input; y output; Tgtf input
function y = fcn(Ego,Tgtf)

Egovx = Ego(4);
Tgtfvx = Tgtf(3);

if Egovx < Tgtfvx+2 && Egovx > Tgtfvx-2
    y = 0;
else
    y = 1;
end

== matlab function Road monito-2024r/rule1_2_5/LatDis ==
  data: Tgtlf input; y output; param input; Ego input; threshlod input
function y = fcn(Tgtlf,param,Ego,threshlod)

tgty = Tgtlf(2);
tgtw = Tgtlf(6);
Egoy = Ego(2);
Egow = param(2);
latdis_p = threshlod(7);

if tgty-0.5*tgtw-Egoy-0.5*Egow > latdis_p
    y = 0;
else
    y = 1;
end

== matlab function Road monito-2024r/rule1_2_6/LatDis ==
  data: Tgtrf input; y output; param input; Ego input; threshlod input
function y = fcn(Tgtrf,param,Ego,threshlod)

tgty = Tgtrf(2);
tgtw = Tgtrf(6);
Egoy = Ego(2);
Egow = param(2);
latdis_p = threshlod(7);

if -tgty-0.5*tgtw-Egoy-0.5*Egow > latdis_p
    y = 0;
else
    y = 1;
end

== matlab function Road monito-2024r/rule1_2_7/LatDis ==
  data: Tgtlr input; y output; param input; Ego input; threshlod input
function y = fcn(Tgtlr,param,Ego,threshlod)

tgty = Tgtlr(2);
tgtw = Tgtlr(6);
Egoy = Ego(2);
Egow = param(2);
latdis_p = threshlod(7);

if tgty-0.5*tgtw-Egoy-0.5*Egow > latdis_p
    y = 0;
else
    y = 1;
end

== matlab function Road monito-2024r/rule1_2_8/LatDis ==
  data: Tgtrr input; y output; param input; Ego input; threshlod input
function y = fcn(Tgtrr,param,Ego,threshlod)

tgty = Tgtrr(2);
tgtw = Tgtrr(6);
Egoy = Ego(2);
Egow = param(2);
latdis_p = threshlod(7);

if -tgty-0.5*tgtw-Egoy-0.5*Egow > latdis_p
    y = 0;
else
    y = 1;
end

== matlab function Road monito-2024r/Subsystem2/MATLAB Function1 ==
  data: u1 input; y output; u1delay input
function y = fcn(u1,u1delay)

if u1 > u1delay % 上升沿，开始换道
    y = 1;
elseif u1 < u1delay % 下降沿，结束换道
    y = -1;
else
    y = 0;
end

== matlab function Road monito-2024r/Enabled Subsystem2/MATLAB Function ==
  data: left input; y output
function y = fcn(left)

type = left(6);
if type == 1 || type == 3 || type == 5
    y = 1;
else
    y = 0;
end

== matlab function Road monito-2024r/Enabled Subsystem3/MATLAB Function ==
  data: left input; y output
function y = fcn(left)

type = left(6);
if type == 1 || type == 3 || type == 4
    y = 1;
else
    y = 0;
end

== matlab function Road monito-2024r/rule44/change_left1/L1 ==
  data: Ego input; Tgt_f input; Tgt_lf input; Tgt_lr input; y1 output; y2 output; y3 output; param input; Threshold input
function [y1,y2,y3] = fcn(Ego,Tgt_f,Tgt_lf,Tgt_lr,param,Threshold)
%%

%参数需求

Tgtx_lr = Tgt_lr(1);             
Tgty_lr = Tgt_lr(2);              
Tgtvx_lr = Tgt_lr(3);
Tgtl_lr = Tgt_lr(5);
Egox = Ego(1);
Egovx = Ego(4);
Egol = param(1);
Ego_fl = param(3);
Tgtx_f = Tgt_f(1);              
Tgty_f = Tgt_f(2);
Tgtvx_f = Tgt_f(3);
Tgtl_f = Tgt_f(5);
Tgtx_lf = Tgt_lf(1);              
Tgty_lf = Tgt_lf(2);
Tgtvx_lf = Tgt_lf(3); 
Tgtl_lf = Tgt_lf(5);
dclmin = Threshold(9) * (Egovx - Tgtvx_lr) + Threshold(10);         %最小换道距离
if dclmin > 50
    dclmin = 50;
elseif dclmin < 0
    dclmin = 0;
else
    dclmin = dclmin;
end
TTCx = Threshold(3);           %安全碰撞时间

%TTC = (Tgtx_f-Egox-0.5*Tgtl_f-Ego_fl)/(Egovx - Tgtvx_f);
%与前车的安全距离判断
if Tgtx_f == 2000 && Tgty_f == 2000       %坐标为2000视为不存在前车
    y1 = 0;   
else
    if Tgtx_f-Egox-0.5*Tgtl_f-Ego_fl < (Egovx - Tgtvx_f) * TTCx 
        y1 = 1;
%     elseif Tgtx_f-Egox-0.5*Tgtl_f-Ego_fl < dclmin %前车暂不考虑车距
%         y1 = 2;
    else
        y1 = 0;
    end
end
%与左前车的安全距离判断
if Tgtx_lf == 2000 && Tgty_lf == 2000     %坐标为2000视为不存在左前车
    y2 = 0;
else
    if Tgtx_lf-Egox-0.5*Tgtl_lf-Ego_fl < (Egovx - Tgtvx_lf) * TTCx 
        y2 = 1;
    else
        y2 = 0;
    end
end
%与左后车的安全距离判断
if Tgtx_lr == 2000 && Tgty_lr == 2000   %坐标为2000视为不存在左后车
    y3 = 0;
else
    if Egox-Tgtx_lr-0.5*Tgtl_lr-(Egol-Ego_fl) < dclmin
        y3 = 3;
    else
        y3 = 0;
    end
end

== matlab function Road monito-2024r/rule44/change_left2/beforerchangelane ==
  data: Tgt_f input; Tgt_r input; y2 output; y3 output; Ego input; param input; Threshold input
function [y2,y3] = fcn(Tgt_f,Tgt_r,Ego,param,Threshold)
%%

%参数需求

Tgtx_r = Tgt_r(1);             
Tgty_r = Tgt_r(2);              
Tgtvx_r = Tgt_r(3);
Tgtl_r = Tgt_r(5);
Egox = Ego(1);
Egovx = Ego(4);
Egol = param(1);
Ego_fl = param(3);
Tgtx_f = Tgt_f(1);              
Tgty_f = Tgt_f(2);
Tgtvx_f = Tgt_f(3); 
Tgtl_f = Tgt_f(5);
dclmin = Threshold(9) * (Egovx - Tgtvx_r) + Threshold(10);         %最小换道距离
if dclmin > 50
    dclmin = 50;
elseif dclmin < 0
    dclmin = 0;
else
    dclmin = dclmin;
end
TTCx = Threshold(3);           %安全碰撞时间

%与前车的安全距离判断
if Tgtx_f == 2000 && Tgty_f == 2000     %坐标为2000视为不存在前车
    y2 = 0;
else
    if Tgtx_f-Egox-0.5*Tgtl_f-Ego_fl < (Egovx - Tgtvx_f) * TTCx 
        y2 = 1;
    else
        y2 = 0;
    end
end
%与后车的安全距离判断
if Tgtx_r == 2000 && Tgty_r == 2000   %坐标为2000视为不存在后车
    y3 = 0;
else
    if Egox-Tgtx_r-0.5*Tgtl_r-(Egol-Ego_fl) < dclmin
        y3 = 3;
    else
        y3 = 0;
    end
end

== matlab function Road monito-2024r/rule44/change_right2/beforerchangelane ==
  data: Tgt_f input; Tgt_r input; y2 output; y3 output; Ego input; param input; Threshold input
function [y2,y3] = fcn(Tgt_f,Tgt_r,Ego,param,Threshold)
%%

%参数需求

Tgtx_r = Tgt_r(1);             
Tgty_r = Tgt_r(2);              
Tgtvx_r = Tgt_r(3);
Tgtl_r = Tgt_r(5);
Egox = Ego(1);
Egovx = Ego(4);
Egol = param(1);
Ego_fl = param(3);
Tgtx_f = Tgt_f(1);              
Tgty_f = Tgt_f(2);
Tgtvx_f = Tgt_f(3); 
Tgtl_f = Tgt_f(5);
dclmin = Threshold(9) * (Egovx - Tgtvx_r) + Threshold(10);         %最小换道距离
if dclmin > 50
    dclmin = 50;
elseif dclmin < 0
    dclmin = 0;
else
    dclmin = dclmin;
end
TTCx = Threshold(3);           %安全碰撞时间

%与前车的安全距离判断
if Tgtx_f == 2000 && Tgty_f == 2000     %坐标为2000视为不存在前车
    y2 = 0;
else
    if Tgtx_f-Egox-0.5*Tgtl_f-Ego_fl < (Egovx - Tgtvx_f) * TTCx 
        y2 = 1;
    else
        y2 = 0;
    end
end
%与后车的安全距离判断
if Tgtx_r == 2000 && Tgty_r == 2000   %坐标为2000视为不存在后车
    y3 = 0;
else
    if Egox-Tgtx_r-0.5*Tgtl_r-(Egol-Ego_fl) < dclmin
        y3 = 3;
    else
        y3 = 0;
    end
end
